simulink model "IPT_th"  (Simulink 7.4)
settings: Solver=FixedStepDiscrete  StartTime=0.0  StopTime=1e6  FixedStep=0.01  RelTol=1e-3
undefined symbols (not defined in the file): IPTc_Gain_ShuntCur, IPTc_Offset_ShuntCur, sigbuilder_block
libraries: Defined_Functionality x1
settings Model: Creator=Administrator  LastModifiedBy=sunsijun
settings DataIOCC: SaveFormat=Structure
settings OptimizationCC: InitFltsAndDblsToZero=on
settings DebuggingCC: InheritedTsInSrcMsg=none  ParameterPrecisionLossMsg=none
settings RTWCC: GenCodeOnly=on

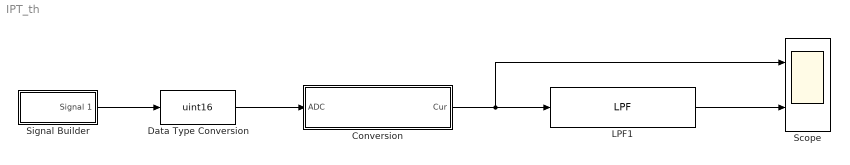
== system IPT_th ==
  Conversion : Subsystem  Description=$Author:Zhao XiangRi$
  Data Type Conversion : DataTypeConversion  OutDataTypeMode=uint16  OutDataType=fixdt(1, 16)  OutScaling=2^0  OutDataTypeStr=uint16
  LPF1 : Defined_Functionality/LPF  SystemSampleTime=-1  filter_gain=IPTc_flter_ShuntCur1
      settings: AttributesFormatString=[FILTER_GAIN=%<filter_gain>]
  Scope : Scope  NumInputPorts=2
      settings: YMin=-5~-5  YMax=5~5
  Signal Builder : Subsystem  Tag=STV Subsys  LoadFcn=sigbuilder_block('load');  StartFcn=sigbuilder_block('start');  StopFcn=sigbuilder_block('stop');  ClipboardFcn=sigbuilder_block('clipboard');  mask(Sigbuilder block){}
      mask help: Sigbuilder GUI
      mask init:
      | if ~strcmp(get_param(bdroot(gcbh),'SimulationStatus'),'stopped') tuvar = sigbuilder_block('maskInit'); end
      settings: CopyFcn=sigbuilder_block('copy');  DeleteFcn=sigbuilder_block('delete');  ModelCloseFcn=sigbuilder_block('modelClose');  PreSaveFcn=sigbuilder_block('preSave');  NameChangeFcn=sigbuilder_block('namechange');  OpenFcn=sigbuilder_block('open',[437.25 199.5 550.5 399.75 ]);  CloseFcn=sigbuilder_block('close');
      mask Display: plot(0,0,100,100,[10,10,40,40,10],[80,20,20,80,80],[40,10],[50,50], [40,27,10],[65,72,56],[40,25,25,10],[28,28,43,43]);
  wires:
  Conversion/1(Cur) -> LPF1/1, Scope/1
  Signal Builder/1(Signal 1) -> Data Type Conversion/1
  LPF1/1 -> Scope/2
  Data Type Conversion/1 -> Conversion/1(ADC)

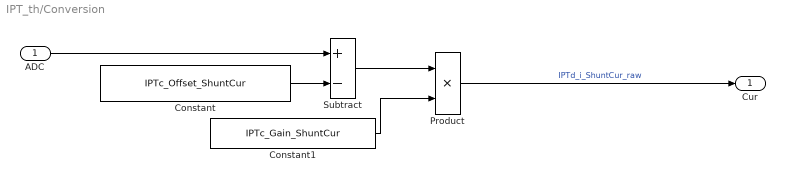
== system IPT_th/Conversion ==
  ADC : Inport  OutDataType=fixdt(1, 16)  OutScaling=2^0
  Constant : Constant  Value=IPTc_Offset_ShuntCur  OutDataTypeMode=single  OutDataType=fixdt(1, 16)  OutScaling=2^0  OutDataTypeStr=single
  Constant1 : Constant  Value=IPTc_Gain_ShuntCur  OutDataTypeMode=single  OutDataType=fixdt(1, 16)  OutScaling=2^0  OutDataTypeStr=single
  Product : Product  OutDataType=fixdt(1, 16)  OutScaling=2^0  RndMeth=Zero
  Subtract : Sum  Inputs=+-  OutDataType=fixdt(1, 16)  OutScaling=2^-10
  Cur : Outport  OutDataType=fixdt(1, 16)  OutScaling=2^0
  wires:
  Product/1 -> Cur/1  "IPTd_i_ShuntCur_raw"
  Constant1/1 -> Product/2
  Constant/1 -> Subtract/2
  Subtract/1 -> Product/1
  ADC/1 -> Subtract/1

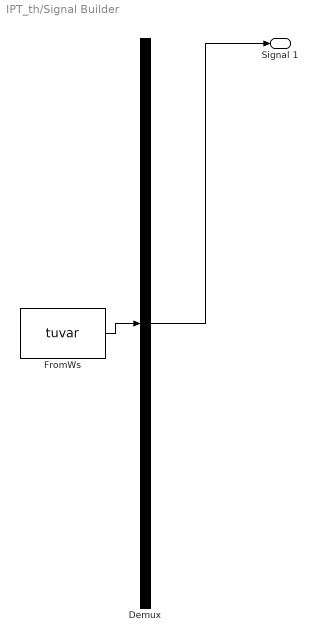
== system IPT_th/Signal Builder ==
  Demux : Demux  Tag=STV Demux  Outputs=1
  FromWs : FromWorkspace  Tag=STV FromWs  VariableName=tuvar  SampleTime=0  SigBuilderData=DataTag0  VnvData=DataTag1
      SigBuilderData=|
      | common.afterFinalStr = 'Extrapolate'
      | common.sampleTime = 0
      | dataSet.timeRange = [0 10]
      | dataSet.name = 'Group 1'
      | sbobj.Groups.Name = 'Group 1'
      | sbobj.Groups.Signals.Name = 'Signal 1'
      | sbobj.Groups.Signals.XData = [0 4 4 4.02 4.02 10]
      | sbobj.Groups.Signals.YData = [32800 32800 6655 6655 32800 32800]
  Signal 1 : Outport  Tag=STV Outport  OutDataType=fixdt(1, 16)  OutScaling=2^0
  wires:
  Demux/1 -> Signal 1/1
  FromWs/1 -> Demux/1
